simulink model "Duty_Cycle_Model"  (R2020a)
settings: Solver=VariableStepAuto  StartTime=0.0  StopTime=0.001  RelTol=1e-3
libraries: powerlib_meascontrol x2, powerlib x1
settings Model: Creator=Ricardo Romero  LastModifiedBy=Ricardo Romero

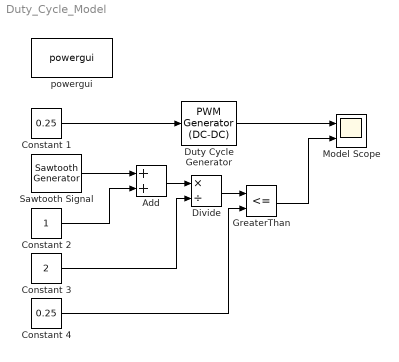
== system Duty_Cycle_Model ==
  Add : Sum
  Constant 1 : Constant  Value=0.25
  Constant 2 : Constant
  Constant 3 : Constant  Value=2
  Constant 4 : Constant  Value=0.25
  Divide : Product  Inputs=*/
  Duty Cycle Generator : powerlib_meascontrol/Pulse & Signal Generators/PWM Generator (DC-DC)  Fsw=5000  Ts=0
  GreaterThan : RelationalOperator  Operator=<=  OutDataTypeStr=boolean  RndMeth=Simplest
  Model Scope : Scope  NumInputPorts=2
  Sawtooth Signal : powerlib_meascontrol/Pulse & Signal Generators/Sawtooth Generator  Freq=5e3  Phase=0  Ts=0
  powergui : powerlib/powergui  Priority=1  SimulationMode=Continuous  SampleTime=50e-6  frequency=60  Iterations=50  frequencyindice=60  Pbase=100e6  ErrMax=1e-4  UnitsV=kV  UnitsW=MW  buscounter=0  FunctionMessages=off  echomessages=off  EnableUseOfTLC=off  CurrentSourceSwitches=off  DisableSnubberDevices=off  DisableRonSwitches=off  DisableVfSwitches=off  DisplayEquations=off  AutomaticDiscreteSolvers=off  SolverType=Tustin/Backward Euler (TBE)  Interpol=off  ExternalGateDelay=off  methode=off  Ts=100  x0status=blocks  SPID=on  SwTol=0  HookPort=off  NonlinearTolerance=1e-4  nMaxIteration=100  ContinueOnMaxIteration=off  RestoreLinks=warning  ResistiveCurrentMeasurement=off  Frange=[0:2:500]  Ylog=off  Xlog=on  ShowGrid=off  save=off  variable=ZData  structure=0  ZoomFFT=off  StartTime=0.0  cycles=1  DisplayStyle=1  fundamental=60  FreqAxis=off  MaxFrequency=1000  frequencyindicesteady=1  RmsSteady=1  display=off
  wires:
  Constant 1/1 -> Duty Cycle Generator/1
  Sawtooth Signal/1 -> Add/1
  Constant 2/1 -> Add/2
  Add/1 -> Divide/1
  Constant 3/1 -> Divide/2
  Divide/1 -> GreaterThan/1
  Constant 4/1 -> GreaterThan/2
  GreaterThan/1 -> Model Scope/2
  Duty Cycle Generator/1 -> Model Scope/1
